simulink model "model"  (R2013b)
settings: Solver=ode45  StartTime=0.0  StopTime=200  RelTol=1e-3
values from neighbouring files (symbols this model uses):
  a45 = 26.02    [simulation.m]
  a90 = 25.31    [simulation.m]
  final_45 = 4    [simulation.m]
  final_90 = 4    [simulation.m]
  init_45 = 0    [simulation.m]
  init_90 = 0    [simulation.m]
  step_45 = 4.81    [simulation.m]
  step_90 = 5.95    [simulation.m]
libraries: cstblocks x2
settings Model: Creator=daniw  LastModifiedBy=daniw

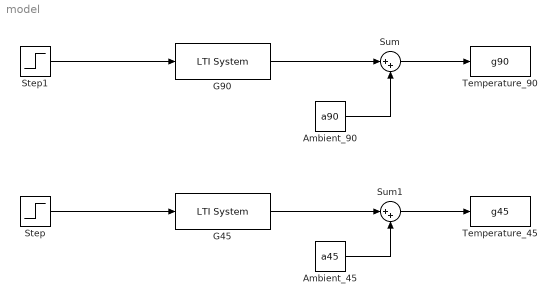
== system model ==
  Ambient_45 : Constant  Value=a45
  Ambient_90 : Constant  Value=a90
  G45 : cstblocks/LTI System  sys=G45  IC=[]
  G90 : cstblocks/LTI System  sys=G90  IC=[]
  Step : Step  Time=step_45  Before=init_45  After=final_45  SampleTime=0
  Step1 : Step  Time=step_90  Before=init_90  After=final_90  SampleTime=0
  Sum : Sum  Inputs=|++
  Sum1 : Sum  Inputs=|++
  Temperature_45 : ToWorkspace  VariableName=g45  SampleTime=-1  SaveFormat=Structure With Time
  Temperature_90 : ToWorkspace  VariableName=g90  SampleTime=-1  SaveFormat=Structure With Time
  wires:
  Step/1 -> G45/1
  Step1/1 -> G90/1
  G90/1 -> Sum/1
  Sum/1 -> Temperature_90/1
  Sum1/1 -> Temperature_45/1
  G45/1 -> Sum1/1
  Ambient_90/1 -> Sum/2
  Ambient_45/1 -> Sum1/2
